simulink model "main"  (R2021a)
settings: Solver=FixedStepAuto  StartTime=0.0  StopTime=10  RelTol=1e-3
InitFcn:
  | load('BusDefinitions.mat')
values from neighbouring files (symbols this model uses):
  A_a_dis = [1  -0.0479044950468; 0  1]    [RSdata_Kalman.mat]
  A_e_dis = [1  0.0479044950468; 0  1]    [RSdata_Kalman.mat]
  A_t_dis = [1  0.00488821378028; 0  1]    [RSdata_Kalman.mat]
  B_a_dis = [-0.000119761237617 0.005]    [RSdata_Kalman.mat]
  B_e_dis = [0.000119761237617 0.005]    [RSdata_Kalman.mat]
  B_t_dis = [1.22205344507e-05 0.005]    [RSdata_Kalman.mat]
  C_a_dis = [1  0; 0  1]    [RSdata_Kalman.mat]
  C_e_dis = [1  0; 0  1]    [RSdata_Kalman.mat]
  C_t_dis = [1 0]    [RSdata_Kalman.mat]
  M = [2.03476350051e-06 9.69056117119e-08 9.69056117119e-08 -1.05662818468e-08 2.03476350051e-06 -9.69056117119e-08 9.69056117119e-08 1.05662818468e-08 2.03476350051e-06 -9.69056117119e-08 -9.69056117119e-08 -1.05662818468e-08 ... (16 elements, 4x4)]    [RSdata_Kalman.mat]
  R_t = 0.00678306479724    [RSdata_Kalman.mat]
undefined symbols (not defined in the file or in its folder): A_r_dis, B_r_dis, C_r_dis, codertarget, Discrete, R_r, Time, Ts, W
libraries: ctrlSharedLib x5
settings Model: ExtModeTrigDuration=80  Creator=tomwh  LastModifiedBy=Liza
settings SolverCC: AlgebraicLoopSolver=TrustRegion
settings OptimizationCC: EnhancedBackFolding=on  PassReuseOutputArgsAs=Individual arguments  ZeroExternalMemoryAtStartup=off  ZeroInternalMemoryAtStartup=off  MaxStackSize=64  OptimizeBlockOrder=speed  DifferentSizesBufferReuse=on  OptimizationCustomize=off  EfficientTunableParamExpr=on
settings DebuggingCC: ParameterTunabilityLossMsg=error  SFMachineParentedDataDiag=warning  ArithmeticOperatorsInVariantConditions=warning
settings HardwareCC: ProdBitPerPointer=32  ProdBitPerSizeT=32  ProdBitPerPtrDiffT=32  ProdLargestAtomicInteger=Long  ProdWordSize=32  ProdHWDeviceType=ARM Compatible->ARM 9  UseEmbeddedCoderFeatures=off
settings SFSimCC: SimUseLocalCustomCode=off  MATLABDynamicMemAlloc=off
settings RTWCC: SystemTargetFile=ert.tlc  HardwareBoard=PARROT Mambo  TemplateMakefile=ert_default_tmf  GenerateReport=on  RTWUseLocalCustomCode=off  Toolchain=Sourcery G++ Lite GNU Toolchain for Drones  LaunchReport=on
settings CodeAppCC: ForceParamTrailComments=on  IgnoreCustomStorageClasses=off  OperatorAnnotations=on  SimulinkDataObjDesc=on  SFDataObjDesc=on  InsertBlockDesc=on
settings ERTTargetCC: MatFileLogging=on  SupportNonInlinedSFcns=on

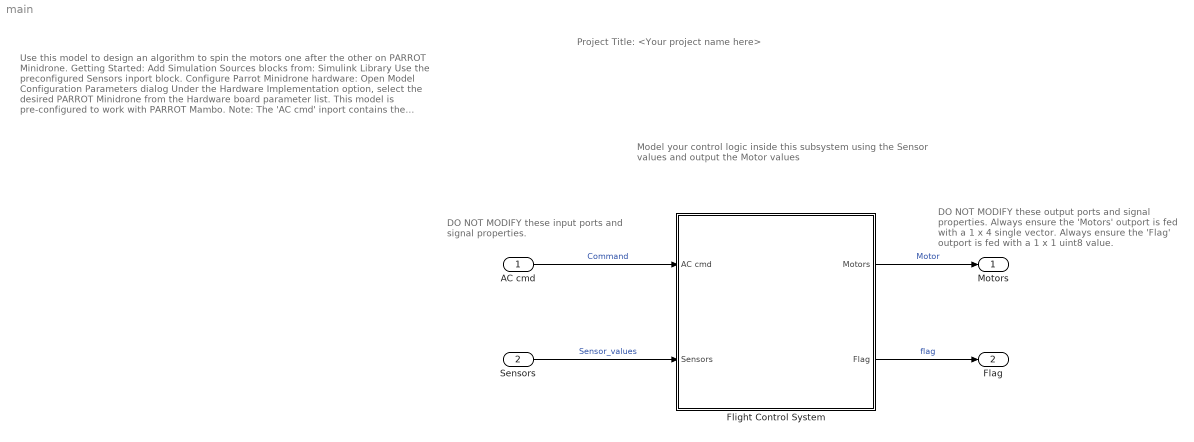
== system main ==
  note: Model your control logic inside this subsystem
      | using the Sensor values and output the
      | Motor values
  note: DO NOT MODIFY these output ports
      | and signal properties.
      |
      |
      |
      | Always ensure the 'Motors' outport
      | is fed with a 1 x 4 single vector.
      |
      |
      |
      |
      |
      | Always ensure the 'Flag' outport is
      | fed with a 1 x 1 uint8 value.
  note: DO NOT MODIFY these input
      | ports and signal properties.
  note: Use this model to design an algorithm to spin the motors one
      | after the other on PARROT Minidrone.
      |
      | Getting Started:
      |
      | Add Simulation Sources blocks from:
      | Simulink Library
      | Use the preconfigured Sensors inport block.
      |
      | Configure Parrot Minidrone hardware:
      |
      | Open Model Configuration Parameters dialog
      |
      | Under the Hardware Implementation option, select the desired
      | PARROT Minidrone from the Hardware board parameter list.
      |
      | This model is pre-configured to work with PARROT Mambo.
      |
      | Note:
      |
      | The 'AC cmd' inport contains the position and orientation
      | reference signals information.
      | The 'Sensors' inport contains data from accelerometer,
      | gyroscope, ultrasonic, pressure and optical flow data.
      | The 'Flag' outport can be used to model an error condition
      | which stops the drone.
      | The 'Motors' outport is fed with the speed values of the 4 motors.
      | Learn more:
      |
      | Simulink Subsystem
      | Simulink Buses
  note: Project Title: <Your project name here>
  AC cmd : Inport  OutDataTypeStr=Bus: CommandBus  BusOutputAsStruct=on
  Sensors : Inport  Port=2  OutDataTypeStr=Bus: SensorsBus  BusOutputAsStruct=on
  Flight Control System : Subsystem  InitFcn=codertarget.parrot.internal.fcsSubsystemCallback(gcb);
  Motors : Outport  OutDataTypeStr=single  PortDimensions=[1 4]  VectorParamsAs1DForOutWhenUnconnected=off
  Flag : Outport  Port=2  OutDataTypeStr=uint8  PortDimensions=1  VectorParamsAs1DForOutWhenUnconnected=off
  wires:
  Flight Control System/1(Motors) -> Motors/1  "Motor"
  AC cmd/1 -> Flight Control System/1(AC cmd)  "Command"
  Sensors/1 -> Flight Control System/2(Sensors)  "Sensor_values"
  Flight Control System/2(Flag) -> Flag/1  "flag"

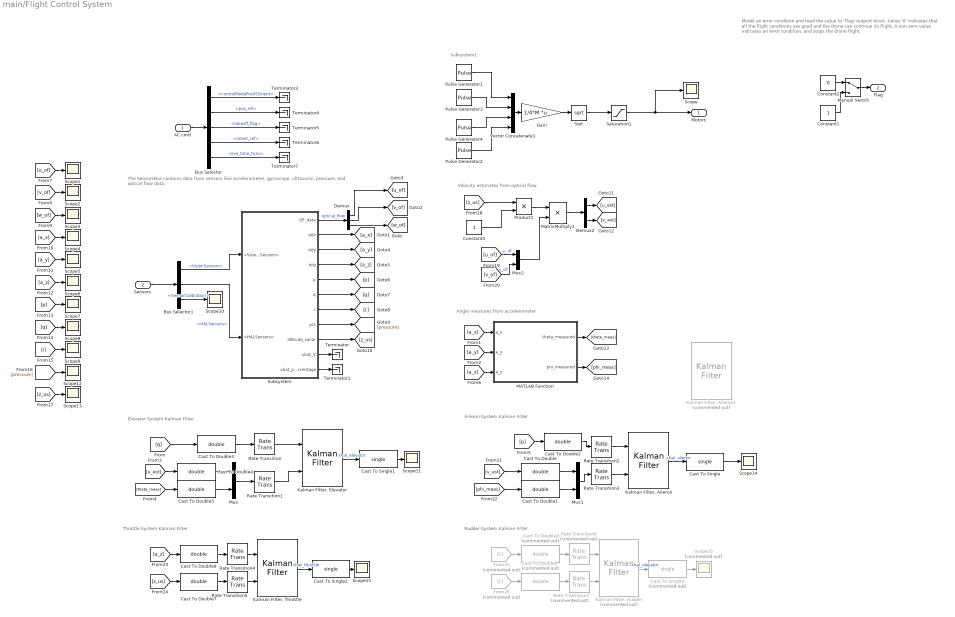
== system main/Flight Control System ==
  note: Elevator System Kalman Filter
  note: Subsystem1
  note: Angle measures from accelerometer
  note: Velocity estimates from optical flow
  note: Model an error condition and feed the value to 'Flag' outport block.
      | Value '0' indicates that all the flight conditions are good and the drone
      | can continue its flight.
      | A non-zero value indicates an error condition, and stops the drone
      | flight.
  note: The SensorsBus contains data from sensors like
      | accelerometer, gyroscope, ultrasonic, pressure,
      | and optical flow data.
  note: Aileron System Kalman Filter
  note: Throttle System Kalman Filter
  note: Rudder System Kalman Filter
  AC cmd : Inport
  Sensors : Inport  Port=2
  Bus Selector : BusSelector  OutputSignals=controlModePosVSOrient,pos_ref,takeoff_flag,orient_ref,live_time_ticks
  Bus Selector1 : BusSelector  OutputSignals=VisionSensors,HALSensors,SensorCalibration
  Cast To Double{,1..7} (8 alike) : DataTypeConversion  OutDataTypeStr=double
  Cast To Double8 : DataTypeConversion  Commented=on  OutDataTypeStr=double
  Cast To Double9 : DataTypeConversion  Commented=on  OutDataTypeStr=double
  Cast To Single : DataTypeConversion  OutDataTypeStr=single
  Cast To Single1 : DataTypeConversion  OutDataTypeStr=single
  Cast To Single2 : DataTypeConversion  OutDataTypeStr=single
  Cast To Single3 : DataTypeConversion  Commented=on  OutDataTypeStr=single
  Constant1 : Constant  OutDataTypeStr=uint8
  Constant2 : Constant  Value=0  OutDataTypeStr=uint8
  Constant3 : Constant
  Demux : Demux  Outputs=3
  Demux2 : Demux  Outputs=2
  From25 : From  Commented=on  GotoTag=r
  From26 : From  Commented=on  GotoTag=r
  Gain : Gain  Gain=1/4*M  Multiplication=Matrix(K*u)
  "Kalman Filter, Aileron" : ctrlSharedLib/Kalman Filter  TimeDomain=Discrete-Time  UseCurrentEstimator=on  ModelSource=Individual A, B, C, D matrices  ModelSourceVariable=ss(0.95,1,1,0,1)  A=A_a_dis  B=B_a_dis  C=C_a_dis  D=[0;0]  NumberOfStates=1  NumberOfInputs=1  NumberOfOutputs=1  InitialEstimateSource=Dialog  X0=[0;0]  P0=10  UseK=off  UseGH=off  NumberOfProcessNoiseInputs=1  G=1  TimeInvariantG=on  H=0  TimeInvariantH=on  Q=Q_a_dis  TimeInvariantQ=on  R=eye(2)  TimeInvariantR=on  N=0  TimeInvariantN=on  AddInputPort=on  AddEnablePort=off  OutputEstimatedY=off  OutputP=off  Ts=1/200
  "Kalman Filter, Aileron1" : ctrlSharedLib/Kalman Filter  Commented=on  TimeDomain=Discrete-Time  UseCurrentEstimator=on  ModelSource=Individual A, B, C, D matrices  ModelSourceVariable=ss(0.95,1,1,0,1)  A=[1 9.8*(1/200); 0 1]  B=[(1/200)^2/2;1/200]  C=eye(2)  D=[0;0]  NumberOfStates=1  NumberOfInputs=1  NumberOfOutputs=1  InitialEstimateSource=Dialog  X0=[0;0]  P0=10  UseK=off  UseGH=off  NumberOfProcessNoiseInputs=1  G=1  TimeInvariantG=on  H=0  TimeInvariantH=on  Q=[(1/200)^2/2;1/200] * [(1/200)^2/2;1/200]'  TimeInvariantQ=on  R=eye(2)  TimeInvariantR=on  N=0  TimeInvariantN=on  AddInputPort=on  AddEnablePort=off  OutputEstimatedY=off  OutputP=off  Ts=1/200
  "Kalman Filter, Elevator" : ctrlSharedLib/Kalman Filter  TimeDomain=Discrete-Time  UseCurrentEstimator=on  ModelSource=Individual A, B, C, D matrices  ModelSourceVariable=ss(0.95,1,1,0,1)  A=A_e_dis  B=B_e_dis  C=C_e_dis  D=[0]  NumberOfStates=1  NumberOfInputs=1  NumberOfOutputs=1  InitialEstimateSource=Dialog  X0=0  P0=10  UseK=off  UseGH=off  NumberOfProcessNoiseInputs=1  G=1  TimeInvariantG=on  H=0  TimeInvariantH=on  Q=Q_e_dis  TimeInvariantQ=on  R=eye(2)  TimeInvariantR=on  N=0  TimeInvariantN=on  AddInputPort=on  AddEnablePort=off  OutputEstimatedY=off  OutputP=off  Ts=1/200
  "Kalman Filter, Rudder" : ctrlSharedLib/Kalman Filter  Commented=on  TimeDomain=Discrete-Time  UseCurrentEstimator=on  ModelSource=Individual A, B, C, D matrices  ModelSourceVariable=ss(0.95,1,1,0,1)  A=A_r_dis  B=B_r_dis  C=C_r_dis  D=[0;0]  NumberOfStates=1  NumberOfInputs=1  NumberOfOutputs=1  InitialEstimateSource=Dialog  X0=0  P0=10  UseK=off  UseGH=off  NumberOfProcessNoiseInputs=1  G=1  TimeInvariantG=on  H=0  TimeInvariantH=on  Q=Q_r_dis  TimeInvariantQ=on  R=R_r  TimeInvariantR=on  N=0  TimeInvariantN=on  AddInputPort=on  AddEnablePort=off  OutputEstimatedY=off  OutputP=off  Ts=1/200
  "Kalman Filter, Throttle" : ctrlSharedLib/Kalman Filter  TimeDomain=Discrete-Time  UseCurrentEstimator=on  ModelSource=Individual A, B, C, D matrices  ModelSourceVariable=ss(0.95,1,1,0,1)  A=A_t_dis  B=B_t_dis  C=C_t_dis  D=0  NumberOfStates=1  NumberOfInputs=1  NumberOfOutputs=1  InitialEstimateSource=Dialog  X0=0  P0=10  UseK=off  UseGH=off  NumberOfProcessNoiseInputs=1  G=1  TimeInvariantG=on  H=0  TimeInvariantH=on  Q=Q_t_dis  TimeInvariantQ=on  R=R_t  TimeInvariantR=on  N=0  TimeInvariantN=on  AddInputPort=on  AddEnablePort=off  OutputEstimatedY=off  OutputP=off  Ts=1/200
  MATLAB Function : MATLAB Function  TreatAsAtomicUnit=on
  Manual Switch : ManualSwitch
  MatrixMultiply1 : Product
  Mux : Mux  Inputs=2
  Mux1 : Mux  Inputs=2
  Mux2 : Mux  Inputs=2
  Product1 : Product
  Pulse Generator1 : DiscretePulseGenerator  Amplitude=W(1)  Period=1600  PulseWidth=400  SampleTime=Ts
  Pulse Generator2 : DiscretePulseGenerator  Amplitude=W(4)  Period=1600  PulseWidth=400  PhaseDelay=1200  SampleTime=Ts
  Pulse Generator3 : DiscretePulseGenerator  Amplitude=W(2)  Period=1600  PulseWidth=400  PhaseDelay=400  SampleTime=Ts
  Pulse Generator4 : DiscretePulseGenerator  Amplitude=W(3)  Period=1600  PulseWidth=400  PhaseDelay=800  SampleTime=Ts
  Rate Transition{,1..5} (6 alike) : RateTransition  OutPortSampleTime=dt
  Rate Transition6 : RateTransition  Commented=on  OutPortSampleTime=dt
  Rate Transition7 : RateTransition  Commented=on  OutPortSampleTime=dt
  Saturation1 : Saturate  UpperLimit=500  LowerLimit=0  OutDataTypeStr=single
  Scope{,1..15} (16 alike) : Scope
  Scope16 : Scope  Commented=on
  Sqrt : Sqrt  SaturateOnIntegerOverflow=on
  Subsystem : Subsystem
  Terminator{,1,3..7} (7 alike) : Terminator
  Vector Concatenate1 : Concatenate  NumInputs=4
  Motors : Outport  VectorParamsAs1DForOutWhenUnconnected=off
  Flag : Outport  Port=2  VectorParamsAs1DForOutWhenUnconnected=off
  wires:
  AC cmd/1 -> Bus Selector/1
  Bus Selector/1 -> Terminator3/1  "<controlModePosVSOrient>"
  Bus Selector/2 -> Terminator4/1  "<pos_ref>"
  Bus Selector/3 -> Terminator5/1  "<takeoff_flag>"
  Bus Selector/4 -> Terminator6/1  "<orient_ref>"
  Bus Selector/5 -> Terminator7/1  "<live_time_ticks>"
  Manual Switch/1 -> Flag/1
  Bus Selector1/1 -> Subsystem/1(<VisionSensors>)  "<VisionSensors>"
  Bus Selector1/3 -> Scope10/1  "<SensorCalibration>"
  Sensors/1 -> Bus Selector1/1
  Bus Selector1/2 -> Subsystem/2(<HALSensors>)  "<HALSensors>"
  Subsystem/10(vbat_V) -> Terminator/1
  Subsystem/11(vbat_percentage) -> Terminator1/1
  Subsystem/2(ddx) -> [a_x]
  Subsystem/1(OF_data) -> Demux/1  "optical_flow"
  Demux/1 -> [u_of]
  Demux/2 -> [v_of]
  Demux/3 -> [w_of]
  Subsystem/3(ddy) -> [a_y]
  Subsystem/4(ddz) -> [a_z]
  Subsystem/5(p) -> [p]
  Subsystem/6(q) -> [q]
  Subsystem/7(r) -> [r]
  Subsystem/8(prs) -> [pressure]
  Subsystem/9(altitude_sonar) -> [z_us]
  [u_of] -> Scope1/1
  [v_of] -> Scope2/1
  [w_of] -> Scope3/1
  [a_x] -> Scope4/1
  [a_y] -> Scope5/1
  [a_z] -> Scope6/1
  [p] -> Scope7/1
  [q] -> Scope8/1
  [r] -> Scope9/1
  [pressure] -> Scope12/1
  [z_us] -> Scope13/1
  Mux2/1 -> MatrixMultiply1/2
  Product1/1 -> MatrixMultiply1/1
  [v_of] -> Mux2/2  "v_of"
  Demux2/2 -> [v_est]
  MatrixMultiply1/1 -> Demux2/1
  Demux2/1 -> [u_est]
  Constant3/1 -> Product1/2
  [u_of] -> Mux2/1  "u_of"
  [z_us] -> Product1/1
  [a_z] -> MATLAB Function/3(a_z)
  [a_x] -> MATLAB Function/1(a_x)
  [a_y] -> MATLAB Function/2(a_y)
  MATLAB Function/1(theta_measured) -> [theta_meas]
  MATLAB Function/2(phi_measured) -> [phi_meas]
  Constant2/1 -> Manual Switch/1
  Constant1/1 -> Manual Switch/2
  Saturation1/1 -> Scope/1, Motors/1
  Pulse Generator3/1 -> Vector Concatenate1/2
  Sqrt/1 -> Saturation1/1
  Gain/1 -> Sqrt/1
  Pulse Generator4/1 -> Vector Concatenate1/3
  Pulse Generator2/1 -> Vector Concatenate1/4
  Vector Concatenate1/1 -> Gain/1
  Pulse Generator1/1 -> Vector Concatenate1/1
  Rate Transition/1 -> "Kalman Filter, Elevator"/1
  Mux/1 -> Rate Transition1/1
  "Kalman Filter, Elevator"/1 -> Cast To Single1/1  "xhat_elevator"
  Rate Transition1/1 -> "Kalman Filter, Elevator"/2
  Mux1/1 -> Rate Transition3/1
  "Kalman Filter, Aileron"/1 -> Cast To Single/1  "xhat_aileron"
  Rate Transition5/1 -> "Kalman Filter, Throttle"/2
  Rate Transition4/1 -> "Kalman Filter, Throttle"/1
  "Kalman Filter, Throttle"/1 -> Cast To Single2/1  "xhat_throttle"
  Rate Transition2/1 -> "Kalman Filter, Aileron"/1
  Rate Transition3/1 -> "Kalman Filter, Aileron"/2
  Cast To Single/1 -> Scope14/1
  [v_est] -> Cast To Double/1
  Cast To Double/1 -> Mux1/1
  [phi_meas] -> Cast To Double1/1
  Cast To Double1/1 -> Mux1/2
  [p] -> Cast To Double2/1
  Cast To Double2/1 -> Rate Transition2/1
  [q] -> Cast To Double3/1
  Cast To Double3/1 -> Rate Transition/1
  [u_est] -> Cast To Double4/1
  [theta_meas] -> Cast To Double5/1
  Cast To Double5/1 -> Mux/2
  Cast To Double4/1 -> Mux/1
  Cast To Single1/1 -> Scope11/1
  Cast To Single2/1 -> Scope15/1
  Cast To Double6/1 -> Rate Transition4/1
  [a_z] -> Cast To Double6/1
  Cast To Double7/1 -> Rate Transition5/1
  [z_us] -> Cast To Double7/1
  "Kalman Filter, Rudder"/1 -> Cast To Single3/1  "xhat_elevator"
  Cast To Double9/1 -> Rate Transition7/1
  Cast To Double8/1 -> Rate Transition6/1
  Rate Transition7/1 -> "Kalman Filter, Rudder"/2
  Cast To Single3/1 -> Scope16/1
  Rate Transition6/1 -> "Kalman Filter, Rudder"/1
  From25/1 -> Cast To Double8/1
  From26/1 -> Cast To Double9/1

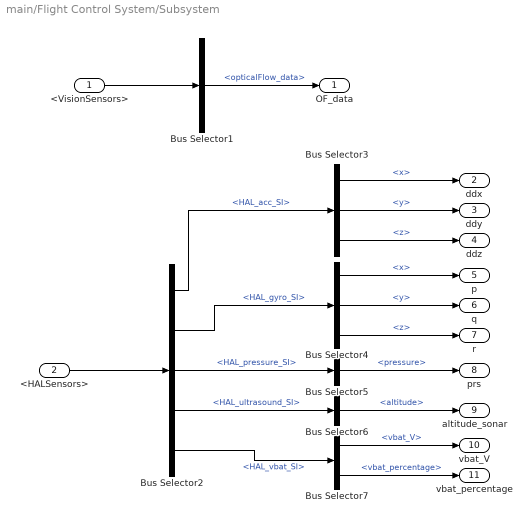
== system main/Flight Control System/Subsystem ==
  <VisionSensors> : Inport
  <HALSensors> : Inport  Port=2
  Bus Selector1 : BusSelector  OutputSignals=opticalFlow_data
  Bus Selector2 : BusSelector  OutputSignals=HAL_acc_SI,HAL_gyro_SI,HAL_pressure_SI,HAL_ultrasound_SI,HAL_vbat_SI
  Bus Selector3 : BusSelector  OutputSignals=x,y,z
  Bus Selector4 : BusSelector  OutputSignals=x,y,z
  Bus Selector5 : BusSelector  OutputSignals=pressure
  Bus Selector6 : BusSelector  OutputSignals=altitude
  Bus Selector7 : BusSelector  OutputSignals=vbat_V,vbat_percentage
  OF_data : Outport  VectorParamsAs1DForOutWhenUnconnected=off
  ddx : Outport  Port=2  VectorParamsAs1DForOutWhenUnconnected=off
  ddy : Outport  Port=3  VectorParamsAs1DForOutWhenUnconnected=off
  ddz : Outport  Port=4  VectorParamsAs1DForOutWhenUnconnected=off
  p : Outport  Port=5  VectorParamsAs1DForOutWhenUnconnected=off
  q : Outport  Port=6  VectorParamsAs1DForOutWhenUnconnected=off
  r : Outport  Port=7  VectorParamsAs1DForOutWhenUnconnected=off
  prs : Outport  Port=8  VectorParamsAs1DForOutWhenUnconnected=off
  altitude_sonar : Outport  Port=9  VectorParamsAs1DForOutWhenUnconnected=off
  vbat_V : Outport  Port=10  VectorParamsAs1DForOutWhenUnconnected=off
  vbat_percentage : Outport  Port=11  VectorParamsAs1DForOutWhenUnconnected=off
  wires:
  <VisionSensors>/1 -> Bus Selector1/1
  <HALSensors>/1 -> Bus Selector2/1
  Bus Selector1/1 -> OF_data/1  "<opticalFlow_data>"
  Bus Selector2/1 -> Bus Selector3/1  "<HAL_acc_SI>"
  Bus Selector2/2 -> Bus Selector4/1  "<HAL_gyro_SI>"
  Bus Selector2/3 -> Bus Selector5/1  "<HAL_pressure_SI>"
  Bus Selector2/4 -> Bus Selector6/1  "<HAL_ultrasound_SI>"
  Bus Selector2/5 -> Bus Selector7/1  "<HAL_vbat_SI>"
  Bus Selector3/1 -> ddx/1  "<x>"
  Bus Selector3/2 -> ddy/1  "<y>"
  Bus Selector3/3 -> ddz/1  "<z>"
  Bus Selector4/2 -> q/1  "<y>"
  Bus Selector4/1 -> p/1  "<x>"
  Bus Selector4/3 -> r/1  "<z>"
  Bus Selector5/1 -> prs/1  "<pressure>"
  Bus Selector6/1 -> altitude_sonar/1  "<altitude>"
  Bus Selector7/1 -> vbat_V/1  "<vbat_V>"
  Bus Selector7/2 -> vbat_percentage/1  "<vbat_percentage>"

== matlab function main/Flight Control System/MATLAB Function ==
  data: a_x input; theta_measured output; a_y input; a_z input; phi_measured output
function [theta_measured,phi_measured]= fcn(a_x,a_y,a_z)
theta_measured = -a_x / sqrt(a_y^2 + a_z^2);
phi_measured = a_y/a_z;
